simulink model "Ex5_2_iv"  (R2022b)
settings: Solver=ode1  StartTime=0.0  StopTime=50  FixedStep=0.001  RelTol=1e-3
settings Model: Creator=super  LastModifiedBy=15043
settings ModelReferenceCC: EnableRefExpFcnMdlSchedulingChecks=on

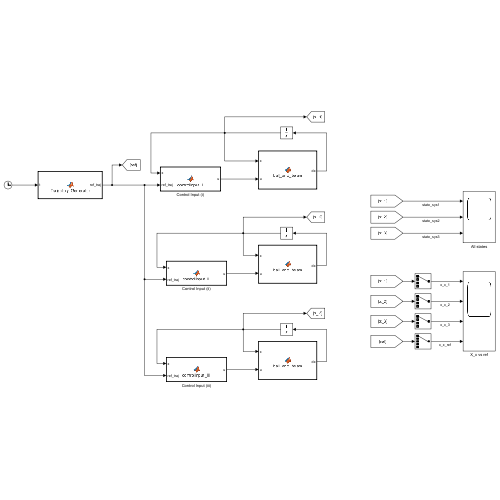
[thumbnail: Simulink's stored preview of the top-level diagram]
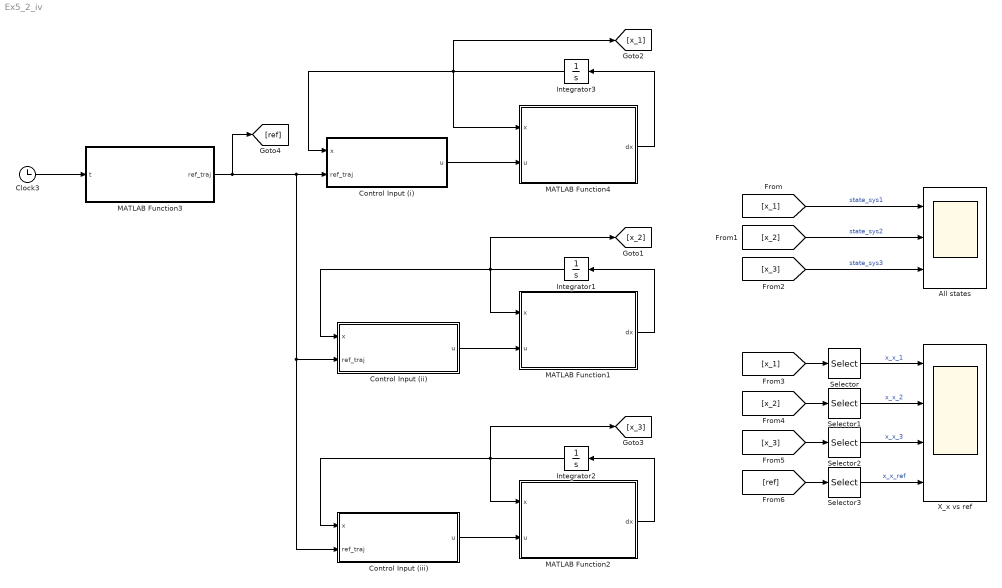
== system Ex5_2_iv ==
  All states : Scope  NumInputPorts=3
  Clock3 : Clock
  Control Input (i) : MATLAB Function  TreatAsAtomicUnit=on
  Control Input (ii) : MATLAB Function  TreatAsAtomicUnit=on
  Control Input (iii) : MATLAB Function  TreatAsAtomicUnit=on
  Integrator1 : Integrator  InitialCondition=[0;0;0;0]
  Integrator2 : Integrator  InitialCondition=[0;0;0;0]
  Integrator3 : Integrator  InitialCondition=[0;0;0;0]
  MATLAB Function1 : MATLAB Function  TreatAsAtomicUnit=on
  MATLAB Function2 : MATLAB Function  TreatAsAtomicUnit=on
  MATLAB Function3 : MATLAB Function  TreatAsAtomicUnit=on
  MATLAB Function4 : MATLAB Function  TreatAsAtomicUnit=on
  Selector : Selector  InputPortWidth=4  IndexOptions=Index vector (dialog)  Indices=[1]  OutputSizes=1
  Selector1 : Selector  InputPortWidth=4  IndexOptions=Index vector (dialog)  Indices=[1]  OutputSizes=1
  Selector2 : Selector  InputPortWidth=4  IndexOptions=Index vector (dialog)  Indices=[1]  OutputSizes=1
  Selector3 : Selector  InputPortWidth=5  IndexOptions=Index vector (dialog)  Indices=[1]  OutputSizes=1
  X_x vs ref : Scope  NumInputPorts=4
  wires:
  Clock3/1 -> MATLAB Function3/1(t)
  MATLAB Function3/1(ref_traj) -> [ref], Control Input (iii)/2(ref_traj), Control Input (ii)/2(ref_traj), Control Input (i)/2(ref_traj)
  Control Input (i)/1(u) -> MATLAB Function4/2(u)
  MATLAB Function4/1(dx) -> Integrator3/1
  Integrator3/1 -> [x_1], MATLAB Function4/1(x), Control Input (i)/1(x)
  [x_1] -> All states/1  "state_sys1"
  Control Input (ii)/1(u) -> MATLAB Function1/2(u)
  MATLAB Function1/1(dx) -> Integrator1/1
  Integrator1/1 -> [x_2], MATLAB Function1/1(x), Control Input (ii)/1(x)
  [x_2] -> All states/2  "state_sys2"
  Control Input (iii)/1(u) -> MATLAB Function2/2(u)
  Integrator2/1 -> Control Input (iii)/1(x), [x_3], MATLAB Function2/1(x)
  MATLAB Function2/1(dx) -> Integrator2/1
  [x_3] -> All states/3  "state_sys3"
  [x_1] -> Selector/1
  [x_2] -> Selector1/1
  [x_3] -> Selector2/1
  [ref] -> Selector3/1
  Selector/1 -> X_x vs ref/1  "x_x_1"
  Selector1/1 -> X_x vs ref/2  "x_x_2"
  Selector2/1 -> X_x vs ref/3  "x_x_3"
  Selector3/1 -> X_x vs ref/4  "x_x_ref"

== matlab function Ex5_2_iv/MATLAB Function1 ==
  data: x input; u input; dx output; par parameter
function dx = ball_and_beam(x,u, par)
    
    % system parameters
    g = par.g;

    % state vector
    x1 = x(1);
    x2 = x(2);
    x3 = x(3);
    x4 = x(4);
         
    % preallocate f vector then put the symbolic expressions calculated
    % from the system model
    f = zeros(4,1);
    f(1) = x2;
    f(2) = (5*x1*x4^2)/7 - (5*g*sin(x3))/7;
    f(3) = x4;
    
    gx = [0; 0; 0; 1];

    dx = f + gx*u;

== matlab function Ex5_2_iv/Control Input (ii) ==
  data: x input; ref_traj input; u output; par parameter
function u = controlInput_II( x, ref_traj, par)
    
    % Coefficients of the hurwitz polynomial
    p0 = par.p(1);
    p1 = par.p(2);
    p2 = par.p(3);
    p3 = par.p(4);
    
    % System parameters
    g = par.g;

    % Reference trajectories and the derivatives from the trajectory
    % generator function
    y_ref       = ref_traj(1);
    y_ref_dot   = ref_traj(2);
    y_ref_ddot  = ref_traj(3);
    y_ref_3dot  = ref_traj(4);
    y_ref_4dot  = ref_traj(5);
    
    % Our state vector X assuming we have access to all the states
    x1 = x(1);  % x_x
    x2 = x(2);  % x_xdot
    x3 = x(3);  % phi_x
    x4 = x(4);  % phi_xdot

    u = -(7*(y_ref_4dot + p2*(y_ref_ddot + (5*g*sin(x3))/7) - p0*(x1 - y_ref) - p1*(x2 - y_ref_dot) + p3*(y_ref_3dot + (5*g*x4*cos(x3))/7) - (5*g*x4^2*sin(x3))/7))/(5*g*cos(x3));

== matlab function Ex5_2_iv/MATLAB Function2 ==
  data: x input; u input; dx output; par parameter
function dx = ball_and_beam(x,u, par)
    
    % system parameters
    g = par.g;

    % state vector
    x1 = x(1);
    x2 = x(2);
    x3 = x(3);
    x4 = x(4);
         
    % preallocate f vector then put the symbolic expressions calculated
    % from the system model
    f = zeros(4,1);
    f(1) = x2;
    f(2) = (5*x1*x4^2)/7 - (5*g*sin(x3))/7;
    f(3) = x4;
    
    gx = [0; 0; 0; 1];

    dx = f + gx*u;

== matlab function Ex5_2_iv/MATLAB Function3 ==
  data: t input; ref_traj output
function ref_traj = Trajectory_Generator(t)

    % Preallocate the reference trajectory and derivatives vector
    ref_traj = zeros(5,1);

    % Symbolic expressions as calculated in remark 5.1
    ref_traj(1) =  cos((pi*t)/2)/25;
    ref_traj(2) = -(pi*sin((pi*t)/2))/50;
    ref_traj(3) = -(pi^2*cos((pi*t)/2))/100;
    ref_traj(4) =  (pi^3*sin((pi*t)/2))/200;
    ref_traj(5) =  (pi^4*cos((pi*t)/2))/400;

== matlab function Ex5_2_iv/Control Input (i) ==
  data: x input; ref_traj input; u output; par parameter
function u = controlInput_I( x, ref_traj, par)
    
    % Coefficients of the hurwitz polynomial
    p0 = par.p(1);
    p1 = par.p(2);
    p2 = par.p(3);
    p3 = par.p(4);
    
    % System parameters
    g = par.g;

    % Reference trajectories and the derivatives from the trajectory
    % generator function
    y_ref       = ref_traj(1);
    y_ref_dot   = ref_traj(2);
    y_ref_ddot  = ref_traj(3);
    y_ref_3dot  = ref_traj(4);
    y_ref_4dot  = ref_traj(5);
    
    % Our state vector X assuming we have access to all the states
    x1 = x(1);  % x_x
    x2 = x(2);  % x_xdot
    x3 = x(3);  % phi_x
    x4 = x(4);  % phi_xdot

    u = (7*(y_ref_4dot + p2*(y_ref_ddot - (5*x1*x4^2)/7 + (5*g*sin(x3))/7) + p3*(y_ref_3dot - (5*x2*x4^2)/7 + (5*g*x4*cos(x3))/7) - p0*(x1 - y_ref) - p1*(x2 - y_ref_dot) - (5*x4^2*(5*x1*x4^2 + 2*g*sin(x3)))/49))/(10*x2*x4 - 5*g*cos(x3));

== matlab function Ex5_2_iv/MATLAB Function4 ==
  data: x input; u input; dx output; par parameter
function dx = ball_and_beam(x,u, par)
    
    % system parameters
    g = par.g;

    % state vector
    x1 = x(1);
    x2 = x(2);
    x3 = x(3);
    x4 = x(4);
         
    % preallocate f vector then put the symbolic expressions calculated
    % from the system model
    f = zeros(4,1);
    f(1) = x2;
    f(2) = (5*x1*x4^2)/7 - (5*g*sin(x3))/7;
    f(3) = x4;
    
    gx = [0; 0; 0; 1];

    dx = f + gx*u;

== matlab function Ex5_2_iv/Control Input (iii) ==
  data: x input; ref_traj input; u output; par parameter
function u = controlInput_III( x, ref_traj, par)
    
    % Coefficients of the hurwitz polynomial
    p0 = par.p(1);
    p1 = par.p(2);
    p2 = par.p(3);
    p3 = par.p(4);
    
    % System parameters
    g = par.g;

    % Reference trajectories and the derivatives from the trajectory
    % generator function
    y_ref       = ref_traj(1);
    y_ref_dot   = ref_traj(2);
    y_ref_ddot  = ref_traj(3);
    y_ref_3dot  = ref_traj(4);
    y_ref_4dot  = ref_traj(5);
    
    % Our state vector X assuming we have access to all the states
    x1 = x(1);  % x_x
    x2 = x(2);  % x_xdot
    x3 = x(3);  % phi_x
    x4 = x(4);  % phi_xdot

    u = -(7*(y_ref_4dot - p0*(x1 - y_ref) - p1*(x2 - y_ref_dot) + p3*(y_ref_3dot + (5*g*x4)/7) + p2*(y_ref_ddot + (5*g*x3)/7)))/(5*g);
